simulink library "gimbalSensorHW_sl"  (R2024b)
settings: Solver=VariableStepAuto  StartTime=0.0  StopTime=10.0  RelTol=1e-3
undefined symbols (not defined in the file): dtSim, gimbalBias, gimbalErrorFlag, gimbalNoisePower
libraries: simulink x1
settings Model: Creator=gilbu
settings RTWCC: GPUComputeCapability=3.5

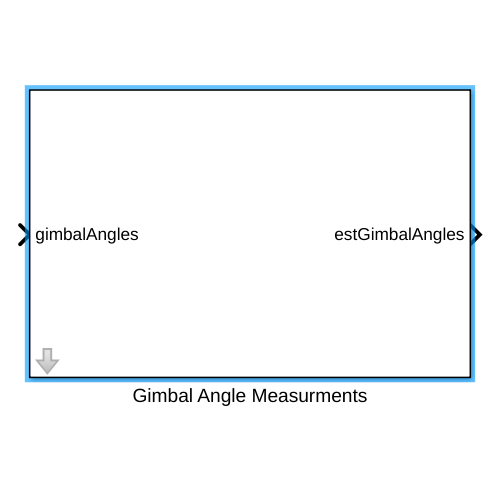
[thumbnail: Simulink's stored preview of the top-level diagram]
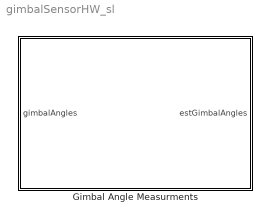
== system gimbalSensorHW_sl ==
  Gimbal Angle Measurments : Subsystem  mask{gimbalErrorFlag=gimbalErrorFlag, gimbalBias=gimbalBias, gimbalNoisePower=gimbalNoisePower}
      mask prompts: gimbalErrorFlag "Gimbal Error Rates <1> [-]"; gimbalBias "Gimbal Rate Bias measurment error <1> [rad/s]"; gimbalNoisePower "White Noise power <1> [rad2/s3]"
      mask DialogControl DescTextVar Prompt: Simulated measurements of gimbal rates of DGCMG. Adds white noise and bias to measuremnets.
      mask DialogControl Control2 Prompt: Gimbal Error Flag equal to one will allow guassian white noise into the angular rate measurements

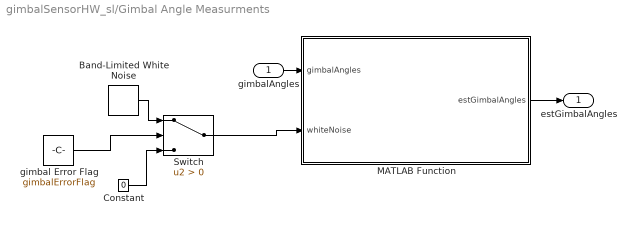
== system gimbalSensorHW_sl/Gimbal Angle Measurments ==
  gimbalAngles : Inport
  Band-Limited White Noise : simulink/Sources/Band-Limited White Noise  Cov=[gimbalNoisePower]  Ts=dtSim  seed=[23341]
  Constant : Constant  Value=0
  MATLAB Function : MATLAB Function  TreatAsAtomicUnit=on
  Switch : Switch  Criteria=u2 > Threshold  SaturateOnIntegerOverflow=off  InputSameDT=off
  gimbal Error Flag : Constant  Value=gimbalErrorFlag
  estGimbalAngles : Outport
  wires:
  Switch/1 -> MATLAB Function/2(whiteNoise)
  gimbalAngles/1 -> MATLAB Function/1(gimbalAngles)
  gimbal Error Flag/1 -> Switch/2
  MATLAB Function/1(estGimbalAngles) -> estGimbalAngles/1
  Band-Limited White Noise/1 -> Switch/1
  Constant/1 -> Switch/3

== matlab function gimbalSensorHW_sl/Gimbal Angle Measurments/MATLAB Function ==
  data: gimbalAngles input double size=8; estGimbalAngles output size=8; whiteNoise input size=1; gimbalBias parameter size=1
% Author: Antonio Gil Buitrago
function estGimbalAngles = gimbalMeasurement( ...
    gimbalAngles,whiteNoise,... %inputs
    gimbalBias...% Parameters
    )
%-------------------------------------------------------------------------------
% Simulated Noise Measurement

estGimbalAngles= gimbalAngles + gimbalBias + whiteNoise;


%-------------------------------------------------------------------------------
end
